simulink model "W10_1_vrx"  (R2024b)
settings: Solver=ode4  StartTime=0.0  StopTime=T_end  FixedStep=Ts_ctrl  RelTol=1e-3
values from neighbouring files (symbols this model uses):
  alloc_mode = 2    [W10_setup.m]
  animate = 1    [W10_setup.m]
  del_max = deg2rad(45)    [W10_setup.m]
  del_rate = deg2rad(30)    [W10_setup.m]
  dp_E0 = 0    [W10_setup.m]
  dp_mode = 1    [W10_setup.m]
  dp_N0 = 0    [W10_setup.m]
  dp_PSI0 = deg2rad(0)    [W10_setup.m]
  dp_ref_on = 1    [W10_setup.m]
  dp_step = [  0    0     0    0 ... (first row only)    [W10_setup.m]
  dp_vmax = [0.5; 0.5; deg2rad(8)]    [W10_setup.m]
  F_max = 500    [W10_setup.m]
  filt_on = 1    [W10_setup.m]
  i_max = [ 200; 200; 400 ]    [W10_setup.m]
  Kd_dp = diag([  110,   110,   200 ])    [W10_setup.m]
  Ki_dp = diag([    5,     5,    16 ])    [W10_setup.m]
  Kp_dp = diag([   50,    50,   160 ])    [W10_setup.m]
  origin_east = -532    [W10_setup.m]
  origin_north = 162    [W10_setup.m]
  T_pinv = pinv(T_e)    [W10_setup.m]    (also in W10_sway_demo.m = evalin('base','T_pinv'))
  tau_del = 0.20    (= 0.2)    [W10_setup.m]
  tau_n = 0.30    (= 0.3)    [W10_setup.m]
  tau_ref = 6    [W10_setup.m]
  Ts_ctrl = 0.05    [W10_setup.m]
  w_filt = 1.20    (= 1.2)    [W10_setup.m]
libraries: ros2lib x9
settings Model: Creator=admin  LastModifiedBy=admin

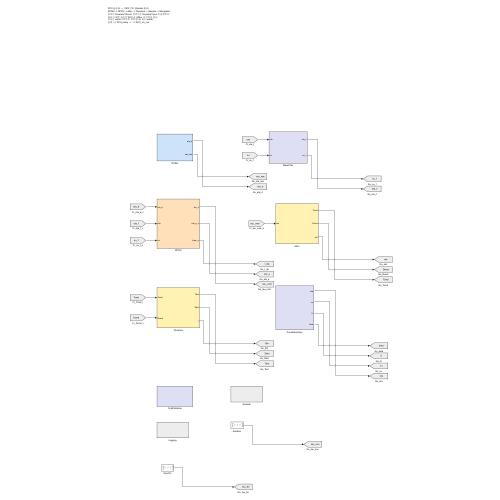
[thumbnail: Simulink's stored preview of the top-level diagram]
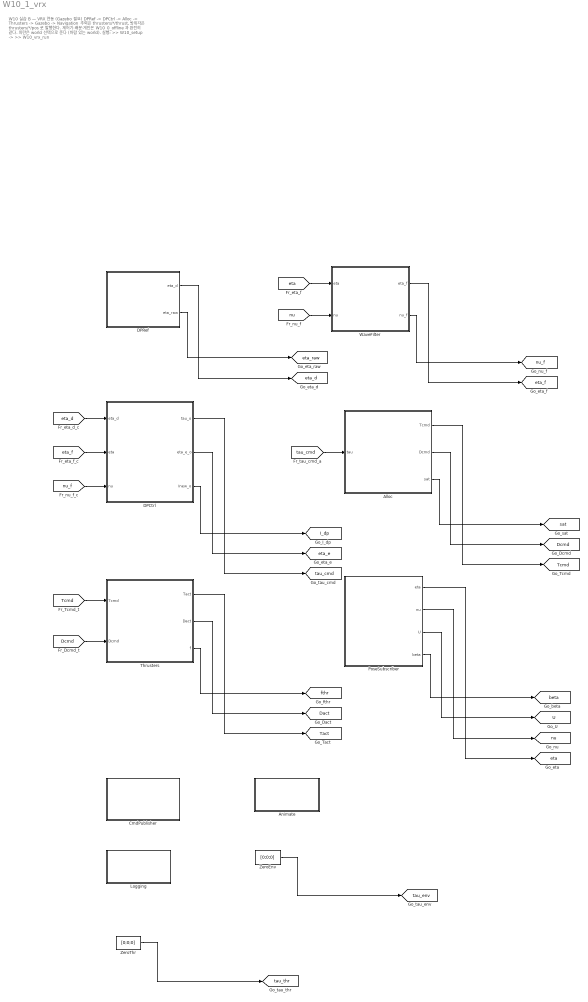
== system W10_1_vrx ==
  note: W10 실습 B  —  VRX 연동 (Gazebo 필요)
      | DPRef -> DPCtrl -> Alloc -> Thrusters -> Gazebo -> Navigation
      | 추력은 thrusters/*/thrust, 방위각은 thrusters/*/pos 로 발행한다.
      | 제어기·배분·게인은 W10_0_offline 과 완전히 같다.
      | 외란은 world 선택으로 준다 (바람 있는 world).
      | 실행: >> W10_setup  ->  >> W10_vrx_run
  Alloc : Subsystem
  Animate : Subsystem
  CmdPublisher : Subsystem
  DPCtrl : Subsystem
  DPRef : Subsystem
  Logging : Subsystem
  PoseSubscriber : Subsystem
  Thrusters : Subsystem
  WaveFilter : Subsystem
  ZeroEnv : Constant  Value=[0;0;0]
  ZeroThr : Constant  Value=[0;0;0]
  tag scope: Dact=global, Dcmd=global, I_dp=global, Tact=global, Tcmd=global, U=global, beta=global, eta=global, eta_d=global, eta_e=global, eta_f=global, eta_raw=global, fthr=global, nu=global, nu_f=global, sat=global, tau_cmd=global, tau_env=global, tau_thr=global
  wires:
  ZeroThr/1 -> [tau_thr]
  ZeroEnv/1 -> [tau_env]
  PoseSubscriber/4(beta) -> [beta]
  PoseSubscriber/3(U) -> [U]
  PoseSubscriber/2(nu) -> [nu]
  PoseSubscriber/1(eta) -> [eta]
  Thrusters/3(f) -> [fthr]
  Thrusters/2(Dact) -> [Dact]
  Thrusters/1(Tact) -> [Tact]
  [Dcmd] -> Thrusters/2(Dcmd)
  [Tcmd] -> Thrusters/1(Tcmd)
  Alloc/3(sat) -> [sat]
  Alloc/2(Dcmd) -> [Dcmd]
  Alloc/1(Tcmd) -> [Tcmd]
  [tau_cmd] -> Alloc/1(tau)
  DPCtrl/3(Inew_o) -> [I_dp]
  DPCtrl/2(eta_e_o) -> [eta_e]
  DPCtrl/1(tau_o) -> [tau_cmd]
  [nu_f] -> DPCtrl/3(nu)
  [eta_f] -> DPCtrl/2(eta)
  [eta_d] -> DPCtrl/1(eta_d)
  WaveFilter/2(nu_f) -> [nu_f]
  WaveFilter/1(eta_f) -> [eta_f]
  [nu] -> WaveFilter/2(nu)
  [eta] -> WaveFilter/1(eta)
  DPRef/2(eta_raw) -> [eta_raw]
  DPRef/1(eta_d) -> [eta_d]

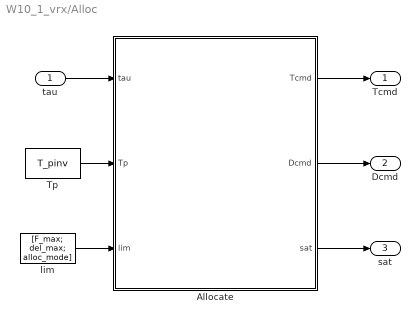
== system W10_1_vrx/Alloc ==
  tau : Inport
  Allocate : MATLAB Function  TreatAsAtomicUnit=on
  Tp : Constant  Value=T_pinv
  lim : Constant  Value=[F_max; del_max; alloc_mode]
  Tcmd : Outport
  Dcmd : Outport  Port=2
  sat : Outport  Port=3
  wires:
  lim/1 -> Allocate/3(lim)
  tau/1 -> Allocate/1(tau)
  Tp/1 -> Allocate/2(Tp)
  Allocate/1(Tcmd) -> Tcmd/1
  Allocate/3(sat) -> sat/1
  Allocate/2(Dcmd) -> Dcmd/1

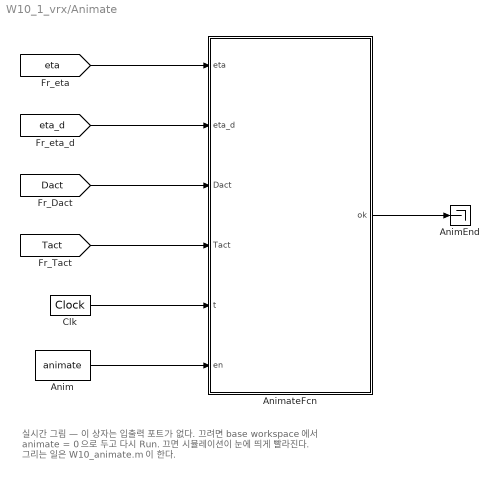
== system W10_1_vrx/Animate ==
  note: 실시간 그림 — 이 상자는 입출력 포트가 없다.
      | 끄려면 base workspace 에서  animate = 0  으로 두고 다시 Run.
      | 끄면 시뮬레이션이 눈에 띄게 빨라진다.
      | 그리는 일은 W10_animate.m 이 한다.
  Anim : Constant  Value=animate
  AnimEnd : Terminator
  AnimateFcn : MATLAB Function  TreatAsAtomicUnit=on
  Clk : DigitalClock  SampleTime=Ts_ctrl
  wires:
  [eta] -> AnimateFcn/1(eta)
  [eta_d] -> AnimateFcn/2(eta_d)
  [Dact] -> AnimateFcn/3(Dact)
  [Tact] -> AnimateFcn/4(Tact)
  Clk/1 -> AnimateFcn/5(t)
  Anim/1 -> AnimateFcn/6(en)
  AnimateFcn/1(ok) -> AnimEnd/1

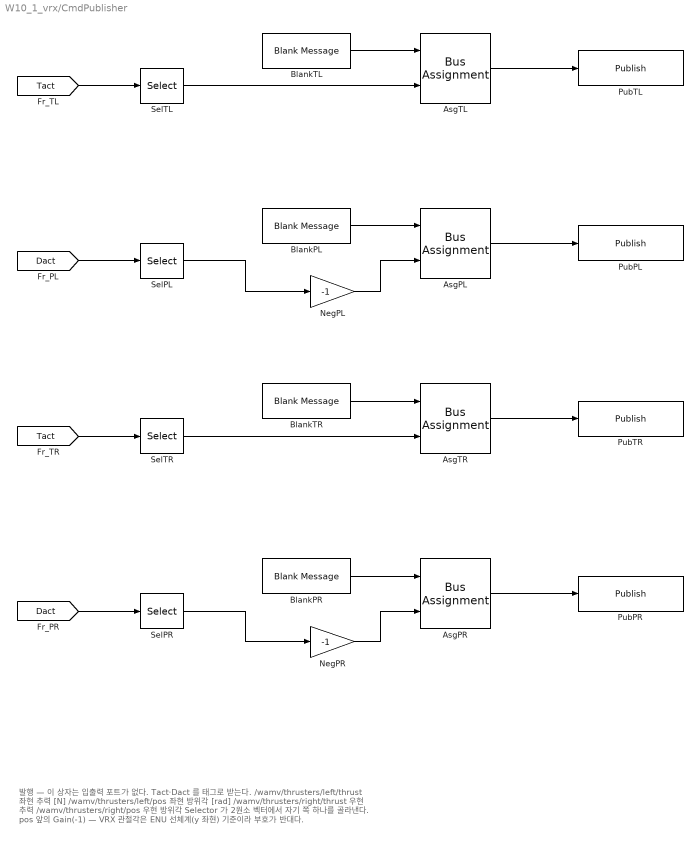
== system W10_1_vrx/CmdPublisher ==
  note: 발행 — 이 상자는 입출력 포트가 없다. Tact·Dact 를 태그로 받는다.
      |   /wamv/thrusters/left/thrust    좌현 추력  [N]
      |   /wamv/thrusters/left/pos       좌현 방위각 [rad]
      |   /wamv/thrusters/right/thrust   우현 추력
      |   /wamv/thrusters/right/pos      우현 방위각
      |
      | Selector 가 2원소 벡터에서 자기 쪽 하나를 골라낸다.
      | pos 앞의 Gain(-1) — VRX 관절각은 ENU 선체계(y 좌현) 기준이라 부호가 반대다.
  AsgPL : BusAssignment  AssignedSignals=data
  AsgPR : BusAssignment  AssignedSignals=data
  AsgTL : BusAssignment  AssignedSignals=data
  AsgTR : BusAssignment  AssignedSignals=data
  BlankPL : ros2lib/Blank Message  messageClass=Message  entityType=std_msgs/Float64  messageType=std_msgs/Float64  SampleTime=Ts_ctrl
  BlankPR : ros2lib/Blank Message  messageClass=Message  entityType=std_msgs/Float64  messageType=std_msgs/Float64  SampleTime=Ts_ctrl
  BlankTL : ros2lib/Blank Message  messageClass=Message  entityType=std_msgs/Float64  messageType=std_msgs/Float64  SampleTime=Ts_ctrl
  BlankTR : ros2lib/Blank Message  messageClass=Message  entityType=std_msgs/Float64  messageType=std_msgs/Float64  SampleTime=Ts_ctrl
  NegPL : Gain  Gain=-1
  NegPR : Gain  Gain=-1
  PubPL : ros2lib/Publish  topicSource=Specify your own  topic=/wamv/thrusters/left/pos  messageType=std_msgs/Float64  QOSHistory=Keep last  QOSDepth=1  QOSReliability=Reliable  QOSDurability=Volatile  QOSDeadline=Inf  QOSLifespan=Inf  QOSLiveliness=Automatic  QOSLeaseDuration=Inf  QOSAvoidROSNamespaceConventions=off
  PubPR : ros2lib/Publish  topicSource=Specify your own  topic=/wamv/thrusters/right/pos  messageType=std_msgs/Float64  QOSHistory=Keep last  QOSDepth=1  QOSReliability=Reliable  QOSDurability=Volatile  QOSDeadline=Inf  QOSLifespan=Inf  QOSLiveliness=Automatic  QOSLeaseDuration=Inf  QOSAvoidROSNamespaceConventions=off
  PubTL : ros2lib/Publish  topicSource=Specify your own  topic=/wamv/thrusters/left/thrust  messageType=std_msgs/Float64  QOSHistory=Keep last  QOSDepth=1  QOSReliability=Reliable  QOSDurability=Volatile  QOSDeadline=Inf  QOSLifespan=Inf  QOSLiveliness=Automatic  QOSLeaseDuration=Inf  QOSAvoidROSNamespaceConventions=off
  PubTR : ros2lib/Publish  topicSource=Specify your own  topic=/wamv/thrusters/right/thrust  messageType=std_msgs/Float64  QOSHistory=Keep last  QOSDepth=1  QOSReliability=Reliable  QOSDurability=Volatile  QOSDeadline=Inf  QOSLifespan=Inf  QOSLiveliness=Automatic  QOSLeaseDuration=Inf  QOSAvoidROSNamespaceConventions=off
  SelPL : Selector  InputPortWidth=2  IndexOptions=Index vector (dialog)  Indices=1  OutputSizes=1
  SelPR : Selector  InputPortWidth=2  IndexOptions=Index vector (dialog)  Indices=2  OutputSizes=1
  SelTL : Selector  InputPortWidth=2  IndexOptions=Index vector (dialog)  Indices=1  OutputSizes=1
  SelTR : Selector  InputPortWidth=2  IndexOptions=Index vector (dialog)  Indices=2  OutputSizes=1
  wires:
  [Tact] -> SelTL/1
  BlankTL/1 -> AsgTL/1
  SelTL/1 -> AsgTL/2
  AsgTL/1 -> PubTL/1
  [Dact] -> SelPL/1
  BlankPL/1 -> AsgPL/1
  SelPL/1 -> NegPL/1
  NegPL/1 -> AsgPL/2
  AsgPL/1 -> PubPL/1
  [Tact] -> SelTR/1
  BlankTR/1 -> AsgTR/1
  SelTR/1 -> AsgTR/2
  AsgTR/1 -> PubTR/1
  [Dact] -> SelPR/1
  BlankPR/1 -> AsgPR/1
  SelPR/1 -> NegPR/1
  NegPR/1 -> AsgPR/2
  AsgPR/1 -> PubPR/1

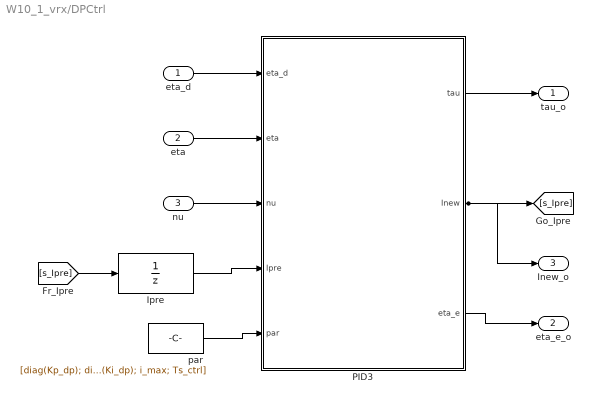
== system W10_1_vrx/DPCtrl ==
  eta_d : Inport
  eta : Inport  Port=2
  nu : Inport  Port=3
  Ipre : UnitDelay  InitialCondition=[0;0;0]  SampleTime=Ts_ctrl  HasFrameUpgradeWarning=on
  PID3 : MATLAB Function  TreatAsAtomicUnit=on
  par : Constant  Value=[diag(Kp_dp); diag(Kd_dp); diag(Ki_dp); i_max; Ts_ctrl]
  tau_o : Outport
  eta_e_o : Outport  Port=2
  Inew_o : Outport  Port=3
  wires:
  PID3/2(Inew) -> Inew_o/1, [s_Ipre]
  [s_Ipre] -> Ipre/1
  eta_d/1 -> PID3/1(eta_d)
  eta/1 -> PID3/2(eta)
  par/1 -> PID3/5(par)
  nu/1 -> PID3/3(nu)
  PID3/1(tau) -> tau_o/1
  Ipre/1 -> PID3/4(Ipre)
  PID3/3(eta_e) -> eta_e_o/1

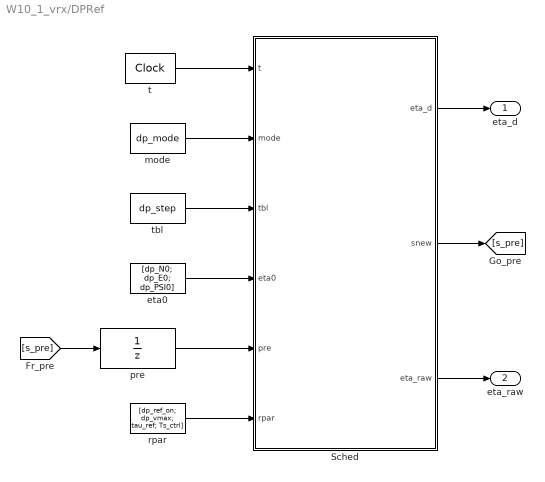
== system W10_1_vrx/DPRef ==
  Sched : MATLAB Function  TreatAsAtomicUnit=on
  eta0 : Constant  Value=[dp_N0; dp_E0; dp_PSI0]
  mode : Constant  Value=dp_mode
  pre : UnitDelay  InitialCondition=[dp_N0; dp_E0; dp_PSI0]  SampleTime=Ts_ctrl  HasFrameUpgradeWarning=on
  rpar : Constant  Value=[dp_ref_on; dp_vmax; tau_ref; Ts_ctrl]
  t : DigitalClock  SampleTime=Ts_ctrl
  tbl : Constant  Value=dp_step
  eta_d : Outport
  eta_raw : Outport  Port=2
  wires:
  [s_pre] -> pre/1
  rpar/1 -> Sched/6(rpar)
  t/1 -> Sched/1(t)
  mode/1 -> Sched/2(mode)
  pre/1 -> Sched/5(pre)
  tbl/1 -> Sched/3(tbl)
  eta0/1 -> Sched/4(eta0)
  Sched/1(eta_d) -> eta_d/1
  Sched/2(snew) -> [s_pre]
  Sched/3(eta_raw) -> eta_raw/1

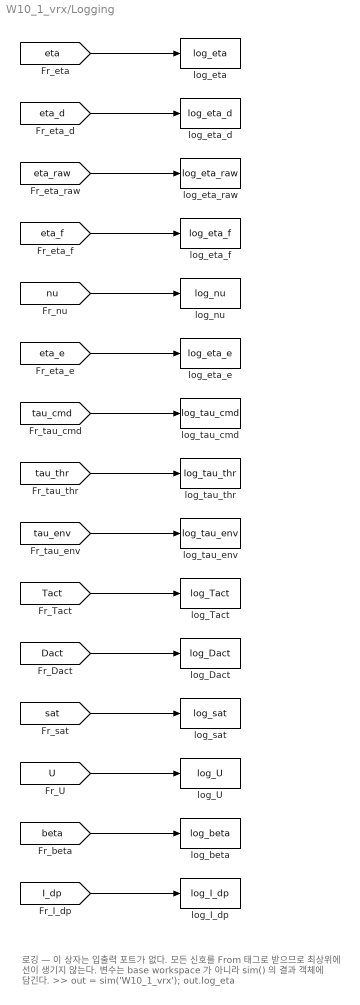
== system W10_1_vrx/Logging ==
  note: 로깅 — 이 상자는 입출력 포트가 없다.
      | 모든 신호를 From 태그로 받으므로 최상위에 선이 생기지 않는다.
      | 변수는 base workspace 가 아니라 sim() 의 결과 객체에 담긴다.
      |   >> out = sim('W10_1_vrx');  out.log_eta
  log_Dact : ToWorkspace  VariableName=log_Dact  SaveFormat=Timeseries  SampleTime=Ts_ctrl
  log_I_dp : ToWorkspace  VariableName=log_I_dp  SaveFormat=Timeseries  SampleTime=Ts_ctrl
  log_Tact : ToWorkspace  VariableName=log_Tact  SaveFormat=Timeseries  SampleTime=Ts_ctrl
  log_U : ToWorkspace  VariableName=log_U  SaveFormat=Timeseries  SampleTime=Ts_ctrl
  log_beta : ToWorkspace  VariableName=log_beta  SaveFormat=Timeseries  SampleTime=Ts_ctrl
  log_eta : ToWorkspace  VariableName=log_eta  SaveFormat=Timeseries  SampleTime=Ts_ctrl
  log_eta_d : ToWorkspace  VariableName=log_eta_d  SaveFormat=Timeseries  SampleTime=Ts_ctrl
  log_eta_e : ToWorkspace  VariableName=log_eta_e  SaveFormat=Timeseries  SampleTime=Ts_ctrl
  log_eta_f : ToWorkspace  VariableName=log_eta_f  SaveFormat=Timeseries  SampleTime=Ts_ctrl
  log_eta_raw : ToWorkspace  VariableName=log_eta_raw  SaveFormat=Timeseries  SampleTime=Ts_ctrl
  log_nu : ToWorkspace  VariableName=log_nu  SaveFormat=Timeseries  SampleTime=Ts_ctrl
  log_sat : ToWorkspace  VariableName=log_sat  SaveFormat=Timeseries  SampleTime=Ts_ctrl
  log_tau_cmd : ToWorkspace  VariableName=log_tau_cmd  SaveFormat=Timeseries  SampleTime=Ts_ctrl
  log_tau_env : ToWorkspace  VariableName=log_tau_env  SaveFormat=Timeseries  SampleTime=Ts_ctrl
  log_tau_thr : ToWorkspace  VariableName=log_tau_thr  SaveFormat=Timeseries  SampleTime=Ts_ctrl
  wires:
  [eta] -> log_eta/1
  [eta_d] -> log_eta_d/1
  [eta_raw] -> log_eta_raw/1
  [eta_f] -> log_eta_f/1
  [nu] -> log_nu/1
  [eta_e] -> log_eta_e/1
  [tau_cmd] -> log_tau_cmd/1
  [tau_thr] -> log_tau_thr/1
  [tau_env] -> log_tau_env/1
  [Tact] -> log_Tact/1
  [Dact] -> log_Dact/1
  [sat] -> log_sat/1
  [U] -> log_U/1
  [beta] -> log_beta/1
  [I_dp] -> log_I_dp/1

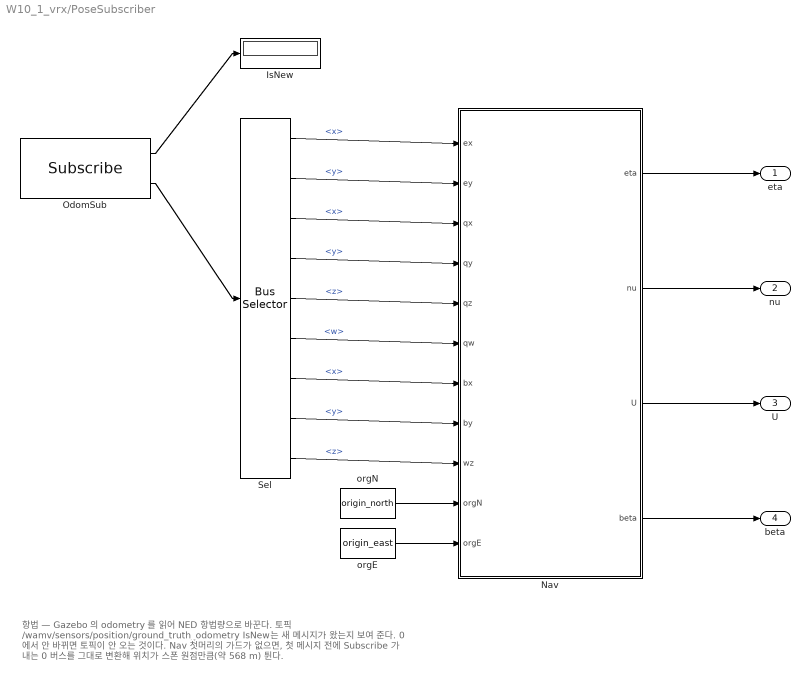
== system W10_1_vrx/PoseSubscriber ==
  note: 항법 — Gazebo 의 odometry 를 읽어 NED 항법량으로 바꾼다.
      |   토픽 /wamv/sensors/position/ground_truth_odometry
      |
      | IsNew 는 새 메시지가 왔는지 보여 준다. 0 에서 안 바뀌면 토픽이 안 오는 것이다.
      | Nav 첫머리의 가드가 없으면, 첫 메시지 전에 Subscribe 가 내는 0 버스를
      | 그대로 변환해 위치가 스폰 원점만큼(약 568 m) 튄다.
  IsNew : Display
  Nav : MATLAB Function  TreatAsAtomicUnit=on
  OdomSub : ros2lib/Subscribe  topicSource=Specify your own  topic=/wamv/sensors/position/ground_truth_odometry  messageType=nav_msgs/Odometry  sampleTime=Ts_ctrl  QOSHistory=Keep last  QOSDepth=1  QOSReliability=Reliable  QOSDurability=Volatile  QOSDeadline=Inf  QOSLifespan=Inf  QOSLiveliness=Automatic  QOSLeaseDuration=Inf  QOSAvoidROSNamespaceConventions=off
  Sel : BusSelector  OutputSignals=pose.pose.position.x,pose.pose.position.y,pose.pose.orientation.x,pose.pose.orientation.y,pose.pose.orientation.z,pose.pose.orientation.w,twist.twist.linear.x,twist.twist.linear.y,twist.twist.angular.z
  orgE : Constant  Value=origin_east
  orgN : Constant  Value=origin_north
  eta : Outport
  nu : Outport  Port=2
  U : Outport  Port=3
  beta : Outport  Port=4
  wires:
  OdomSub/1 -> IsNew/1
  OdomSub/2 -> Sel/1
  Sel/1 -> Nav/1(ex)  "<x>"
  Sel/2 -> Nav/2(ey)  "<y>"
  Sel/3 -> Nav/3(qx)  "<x>"
  Sel/4 -> Nav/4(qy)  "<y>"
  Sel/5 -> Nav/5(qz)  "<z>"
  Sel/6 -> Nav/6(qw)  "<w>"
  Sel/7 -> Nav/7(bx)  "<x>"
  Sel/8 -> Nav/8(by)  "<y>"
  Sel/9 -> Nav/9(wz)  "<z>"
  orgN/1 -> Nav/10(orgN)
  orgE/1 -> Nav/11(orgE)
  Nav/1(eta) -> eta/1
  Nav/2(nu) -> nu/1
  Nav/3(U) -> U/1
  Nav/4(beta) -> beta/1

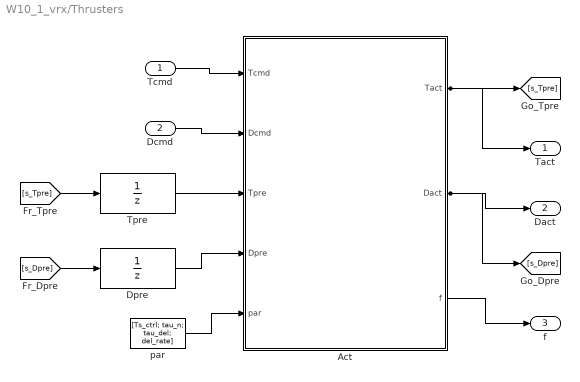
== system W10_1_vrx/Thrusters ==
  Tcmd : Inport
  Dcmd : Inport  Port=2
  Act : MATLAB Function  TreatAsAtomicUnit=on
  Dpre : UnitDelay  InitialCondition=[0;0]  SampleTime=Ts_ctrl  HasFrameUpgradeWarning=on
  Tpre : UnitDelay  InitialCondition=[0;0]  SampleTime=Ts_ctrl  HasFrameUpgradeWarning=on
  par : Constant  Value=[Ts_ctrl; tau_n; tau_del; del_rate]
  Tact : Outport
  Dact : Outport  Port=2
  f : Outport  Port=3
  wires:
  Tpre/1 -> Act/3(Tpre)
  Dcmd/1 -> Act/2(Dcmd)
  [s_Tpre] -> Tpre/1
  par/1 -> Act/5(par)
  Tcmd/1 -> Act/1(Tcmd)
  [s_Dpre] -> Dpre/1
  Dpre/1 -> Act/4(Dpre)
  Act/1(Tact) -> Tact/1, [s_Tpre]
  Act/2(Dact) -> Dact/1, [s_Dpre]
  Act/3(f) -> f/1

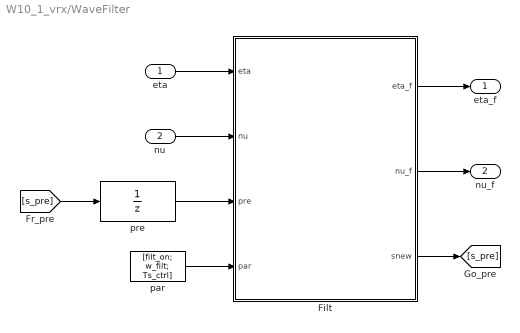
== system W10_1_vrx/WaveFilter ==
  eta : Inport
  nu : Inport  Port=2
  Filt : MATLAB Function  TreatAsAtomicUnit=on
  par : Constant  Value=[filt_on; w_filt; Ts_ctrl]
  pre : UnitDelay  InitialCondition=[0;0;0;0;0;0]  SampleTime=Ts_ctrl  HasFrameUpgradeWarning=on
  eta_f : Outport
  nu_f : Outport  Port=2
  wires:
  Filt/3(snew) -> [s_pre]
  Filt/2(nu_f) -> nu_f/1
  [s_pre] -> pre/1
  eta/1 -> Filt/1(eta)
  nu/1 -> Filt/2(nu)
  pre/1 -> Filt/3(pre)
  par/1 -> Filt/4(par)
  Filt/1(eta_f) -> eta_f/1

== matlab function W10_1_vrx/Animate/AnimateFcn ==
  data: eta input; ok output; eta_d input; Dact input; Tact input; t input; en input
function ok = AnimateFcn(eta, eta_d, Dact, Tact, t, en)
%#codegen
% Live plot while the model runs. A MATLAB Function block cannot
% plot, so the drawing function is declared extrinsic: Simulink
% calls plain MATLAB instead of generating code for it.
coder.extrinsic('W10_animate');
ok = 1;
if en > 0.5
    W10_animate(eta, eta_d, Dact, Tact, t);
end

== matlab function W10_1_vrx/WaveFilter/Filt ==
  data: eta input; eta_f output; nu input; pre input; par input; nu_f output; snew output
function [eta_f, nu_f, snew] = Filt(eta, nu, pre, par)
%#codegen
% Wave filtering for dynamic positioning.
%
% First order wave loads make the vessel oscillate at the wave
% frequency. That motion cannot be counteracted — trying to do so
% only wears out the thrusters. A DP system therefore feeds the
% controller with the LOW FREQUENCY part of the motion only.
% Fossen (2011) 11.4.1 uses a passive observer; here a first order
% low pass with a cut-off well below the wave frequency is enough to
% show the effect.
%
% par = [on; wf; Ts]

on = par(1); wf = par(2); Ts = par(3);
z  = [eta; nu];
if on < 0.5
    eta_f = eta;  nu_f = nu;  snew = z;
    return
end
a = Ts*wf/(1 + Ts*wf);
snew = pre + a*(z - pre);
% heading must be filtered on the difference, not the raw angle
d3 = atan2(sin(eta(3) - pre(3)), cos(eta(3) - pre(3)));
snew(3) = pre(3) + a*d3;
snew(3) = atan2(sin(snew(3)), cos(snew(3)));
eta_f = snew(1:3);
nu_f  = snew(4:6);

== matlab function W10_1_vrx/DPRef/Sched ==
  data: t input; eta_d output; mode input; tbl input; eta0 input; pre input; rpar input; snew output; eta_raw output
function [eta_d, snew, eta_raw] = Sched(t, mode, tbl, eta0, pre, rpar)
%#codegen
% DP setpoint scheduler and REFERENCE MODEL.
%
%   mode 0 : hold the initial setpoint
%   mode 1 : step through the table  [t  N  E  psi_deg]
%
% A raw step demand is never given to a DP controller. The vessel
% cannot move at any speed, so a step makes the controller ask for a
% force the thrusters cannot deliver, and the loop saturates.
% A reference model turns the step into a feasible trajectory. Here a
% saturated proportional law is used:
%     v = (eta_raw - eta_d)/tau_ref,   |v| <= v_max
% Far from the target the setpoint moves at the constant speed v_max;
% close to it the approach becomes exponential with time constant
% tau_ref, so there is no corner at arrival.
% Fossen (2011) calls this the reference model; every DP system has
% one.
%
% rpar = [on; vN; vE; vPsi; tau_ref; Ts]

eta_raw = eta0;
if mode > 0.5
    n = size(tbl,1);
    for i = 1:n
        if t >= tbl(i,1)
            eta_raw = [tbl(i,2); tbl(i,3); tbl(i,4)*pi/180];
        end
    end
end

if rpar(1) < 0.5
    eta_d = eta_raw;  snew = eta_raw;
    return
end

vmax = rpar(2:4);  tr = rpar(5);  Ts = rpar(6);
snew = pre;
for i = 1:3
    d = eta_raw(i) - pre(i);
    if i == 3, d = atan2(sin(d), cos(d)); end
    v = d/tr;
    if v >  vmax(i), v =  vmax(i); end
    if v < -vmax(i), v = -vmax(i); end
    snew(i) = pre(i) + v*Ts;
end
snew(3) = atan2(sin(snew(3)), cos(snew(3)));
eta_d = snew;

== matlab function W10_1_vrx/DPCtrl/PID3 ==
  data: eta_d input; tau output; eta input; nu input; Ipre input; par input; Inew output; eta_e output
function [tau, Inew, eta_e] = PID3(eta_d, eta, nu, Ipre, par)
%#codegen
% 3-DOF dynamic positioning controller (Fossen 2011, 12.2.10).
%
%   eta   = [N; E; psi]      position and heading in NED
%   nu    = [u; v; r]        velocity in BODY
%   tau   = -J(psi)' * (Kp*eta_e + Ki*I) - Kd*nu
%
% The transpose of the rotation matrix turns a NED position error into
% a BODY force. Damping is taken on BODY velocity directly, so no
% derivative of the error is needed (same idea as the P-D heading
% controller of week 7).
%
% par = [Kp(1:3); Kd(1:3); Ki(1:3); imax(1:3); Ts]

Kp = par(1:3);  Kd = par(4:6);  Ki = par(7:9);
im = par(10:12); Ts = par(13);

e = eta - eta_d;
e(3) = atan2(sin(e(3)), cos(e(3)));      % smallest signed angle

psi = eta(3);
J = [ cos(psi), -sin(psi), 0;
      sin(psi),  cos(psi), 0;
             0,         0, 1];

% integral state with clamping (anti-windup)
Inew = Ipre + Ts*e;
for i = 1:3
    lim = im(i)/max(Ki(i), 1e-9);
    if Inew(i) >  lim, Inew(i) =  lim; end
    if Inew(i) < -lim, Inew(i) = -lim; end
end

tau = -J' * ( Kp.*e + Ki.*Inew ) - Kd.*nu;
eta_e = e;

== matlab function W10_1_vrx/Alloc/Allocate ==
  data: tau input; Tcmd output; Tp input; lim input; Dcmd output; sat output
function [Tcmd, Dcmd, sat] = Allocate(tau, Tp, lim)
%#codegen
% Thrust allocation for two azimuth (rotatable) thrusters.
% Fossen (2011) 12.3.4 — constrained control allocation for azimuth
% thrusters, solved with the EXTENDED THRUST VECTOR.
%
% Step 1  f = pinv(T_e) * tau       f = [FxL FyL FxR FyR]'
%         Because the thruster force is written in Cartesian components,
%         T_e is CONSTANT and its pseudo-inverse can be precomputed.
%         There is no singular configuration to worry about.
%
% Step 2  Cartesian -> polar   T = |f_i|,  delta = atan2(Fy, Fx)
%
% Step 3  map the demand into the mechanical sector |delta| <= 45 deg
%           |d| <=  45  : use as is
%           |d| >  135  : REVERSE thrust, d -> d -+ 180
%           otherwise   : dead zone, no thrust can be produced
%
% Step 4  saturate the magnitude at F_max
%
% lim = [F_max; delta_max; mode]
%   mode 1 : dead zone   — demands inside the forbidden sector are
%            dropped. Simple, but the realised tau is then wrong.
%   mode 2 : clamp       — the angle is pushed to the nearest sector
%            edge and the magnitude is scaled by cos of the angle
%            error, so the useful component is kept.

f = Tp * tau;
Fmax = lim(1);  dmax = lim(2);  mode = lim(3);

Tcmd = zeros(2,1);  Dcmd = zeros(2,1);  sat = 0;
for i = 1:2
    fx = f(2*i-1);  fy = f(2*i);
    Ti = sqrt(fx*fx + fy*fy);
    di = atan2(fy, fx);
    ad = abs(di);
    if ad <= dmax
        To = Ti;   Do = di;
    elseif ad >= pi - dmax
        To = -Ti;  Do = di - sign(di)*pi;    % reverse thrust
    elseif mode < 1.5
        To = 0;    Do = 0;                   % dead zone
        sat = sat + 1;
    else
        % clamp to the nearest edge of the reachable sector
        if ad <= pi/2
            Do = sign(di)*dmax;      To =  Ti*cos(ad - dmax);
        else
            Do = -sign(di)*dmax;        To = -Ti*cos(pi - dmax - ad);
            Do = atan2(sin(Do), cos(Do));
        end
        sat = sat + 1;
    end
    if To >  Fmax, To =  Fmax; sat = sat + 1; end
    if To < -Fmax, To = -Fmax; sat = sat + 1; end
    Tcmd(i) = To;  Dcmd(i) = Do;
end

== matlab function W10_1_vrx/Thrusters/Act ==
  data: Tcmd input; Tact output; Dcmd input; Tpre input; Dpre input; par input; Dact output; f output
function [Tact, Dact, f] = Act(Tcmd, Dcmd, Tpre, Dpre, par)
%#codegen
% Actuator dynamics of an azimuth thruster.
%   thrust  : first order lag, time constant tau_n
%   azimuth : first order lag (tau_del) whose angular RATE is capped
%             at rate_max. A real pod cannot snap to a new angle.
% par = [Ts; tau_n; tau_del; rate_max]

Ts = par(1); tn = par(2); td = par(3); rmax = par(4);

Tact = Tpre + (Ts/tn)*(Tcmd - Tpre);

Dact = Dpre;
for i = 1:2
    dd = Dcmd(i) - Dpre(i);
    dd = atan2(sin(dd), cos(dd));           % shortest way round
    step = (Ts/td)*dd;                      % first order lag ...
    lim  = rmax*Ts;                         % ... whose RATE is capped
    if step >  lim, step =  lim; end
    if step < -lim, step = -lim; end
    Dact(i) = Dpre(i) + step;
end

% back to Cartesian components in BODY
f = [ Tact(1)*cos(Dact(1));
      Tact(1)*sin(Dact(1));
      Tact(2)*cos(Dact(2));
      Tact(2)*sin(Dact(2)) ];

== matlab function W10_1_vrx/PoseSubscriber/Nav ==
  data: ex input; eta output; ey input; qx input; qy input; qz input; qw input; bx input; by input; wz input; orgN input; orgE input; nu output; U output; beta output
function [eta, nu, U, beta] = Nav(ex, ey, qx, qy, qz, qw, bx, by, wz, orgN, orgE)
%#codegen
% Gazebo/ROS uses ENU with a body frame of x-forward, y-LEFT, z-UP.
% Marine control uses NED with x-forward, y-STARBOARD, z-DOWN.
% 첫 메시지가 도착하기 전에는 Subscribe 가 0 으로 채운 버스를 낸다.
% 그대로 쓰면 위치가 스폰 원점만큼(약 568 m) 튀어 로그 첫 점이 망가진다.
if ex == 0 && ey == 0
    eta = zeros(3,1); nu = zeros(3,1); U = 0; beta = 0;
    return
end
pn = ey - orgN;
pe = ex - orgE;
yaw_enu = atan2(2*(qw*qz + qx*qy), 1 - 2*(qy*qy + qz*qz));
p   = pi/2 - yaw_enu;
psi = atan2(sin(p), cos(p));
u = bx;  v = -by;  r = -wz;
eta  = [pn; pe; psi];
nu   = [u; v; r];
U    = sqrt(u*u + v*v);
beta = atan2(v, u);
